simulink model "sim_magne_lev"  (R2021a)
settings: Solver=FixedStepAuto  StartTime=0.0  StopTime=15.0  RelTol=1e-3
undefined symbols (not defined in the file or in its folder): National_Instruments, PCIe
libraries: sldrtlib x2
settings Model: SimulationMode=external  Creator=磁気浮上  LastModifiedBy=磁気浮上
settings SolverCC: AlgebraicLoopSolver=TrustRegion  DecoupledContinuousIntegration=on  MinimalZcImpactIntegration=on
settings DataIOCC: ReturnWorkspaceOutputs=off
settings DebuggingCC: SFMachineParentedDataDiag=warning  ArithmeticOperatorsInVariantConditions=warning
settings SFSimCC: SimUseLocalCustomCode=off  CustomCodeUndefinedFunction=UseInterfaceOnly
settings RTWCC: Description=Simulink Desktop Real-Time  SystemTargetFile=sldrt.tlc  TemplateMakefile=sldrt.tmf  RTWUseLocalCustomCode=off  RTWCompilerOptimization=on
settings CodeAppCC: MaxIdLength=95
settings SimulinkDesktopRealTimeCC: TargetPreCompLibLocation=C:\Program Files\MATLAB\R2021a\toolbox\sldrt\lib\win64

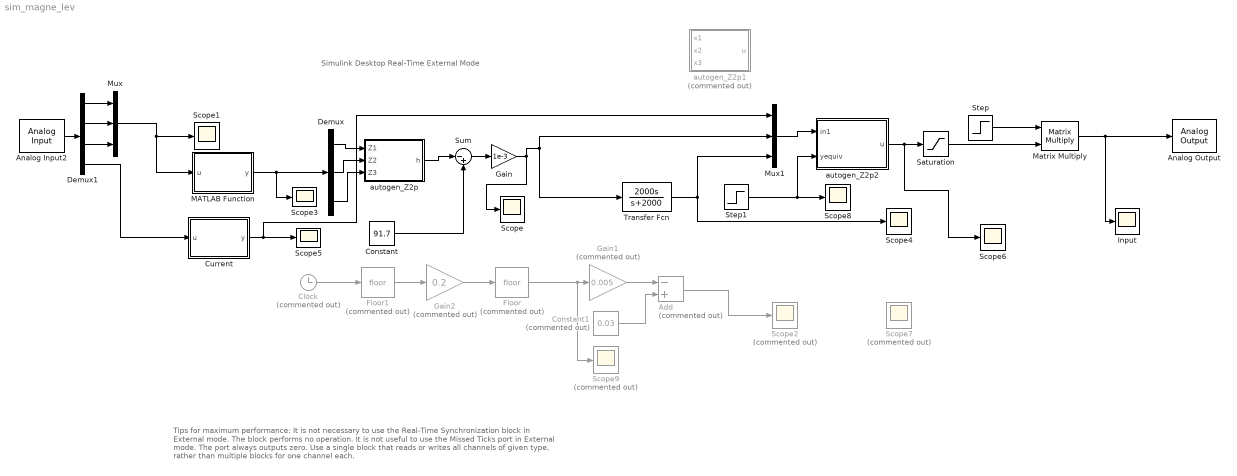
== system sim_magne_lev ==
  note: Simulink Desktop Real-Time External Mode
  note: Tips for maximum performance:
      |
      | It is not necessary to use the Real-Time Synchronization block in External mode. The block performs no operation.
      | It is not useful to use the Missed Ticks port in External mode. The port always outputs zero.
      | Use a single block that reads or writes all channels of given type, rather than multiple blocks for one channel each.
  Add : Sum  Commented=on  Inputs=-+
  Analog Input2 : sldrtlib/Analog Input  SampleTime=0.001  MaxMissedTicks=10  ShowMissedTicks=off  YieldWhenWaiting=off  DrvName=National_Instruments/PCIe-6361  DrvAddress=4294967295  DrvOptions=[0 0 0 0 0 0 0]  Channels=[1 2 3 5]  RangeMode=1  VoltRange=1  DataType=1
      settings: AttributesFormatString=National Instruments\nPCIe-6361 [auto]
  Analog Output : sldrtlib/Analog Output  SampleTime=0.001  MaxMissedTicks=10  ShowMissedTicks=off  YieldWhenWaiting=off  DrvName=National_Instruments/PCIe-6361  DrvAddress=4294967295  DrvOptions=[0 0 0 0 0 0 0]  Channels=1  RangeMode=1  VoltRange=1  InitialValue=[]  FinalValue=[]
      settings: AttributesFormatString=National Instruments\nPCIe-6361 [auto]
  Clock : Clock  Commented=on
  Constant : Constant  Value=91.7
  Constant1 : Constant  Commented=on  Value=0.03
  Current : MATLAB Function  TreatAsAtomicUnit=on
  Demux : Demux  Outputs=3
  Demux1 : Demux
  Floor : Rounding  Commented=on
  Floor1 : Rounding  Commented=on
  Gain : Gain  Gain=1e-3
  Gain1 : Gain  Commented=on  Gain=0.005
  Gain2 : Gain  Commented=on  Gain=0.2
  Input : Scope
  MATLAB Function : MATLAB Function  TreatAsAtomicUnit=on
  Matrix Multiply : Product  Multiplication=Matrix(*)
  Mux : Mux  Inputs=3
  Mux1 : Mux  Inputs=3
  Saturation : Saturate  UpperLimit=10  LowerLimit=-10
  Scope{,1,3..6,8} (7 alike) : Scope
  Scope2 : Scope  Commented=on
  Scope7 : Scope  Commented=on
  Scope9 : Scope  Commented=on
  Step : Step  Time=10  Before=1  After=0  SampleTime=0
  Step1 : Step  Time=5  Before=0.01  After=0.005  SampleTime=0
  Sum : Sum  Inputs=|-+
  Transfer Fcn : TransferFcn  Numerator=[2000 0]  Denominator=[1 2000]
  autogen_Z2p : MATLAB Function  TreatAsAtomicUnit=on
  autogen_Z2p1 : MATLAB Function  Commented=on  TreatAsAtomicUnit=on
  autogen_Z2p2 : MATLAB Function  TreatAsAtomicUnit=on
  wires:
  Step/1 -> Matrix Multiply/1
  Constant/1 -> Sum/2
  autogen_Z2p/1(h) -> Sum/1
  Matrix Multiply/1 -> Input/1, Analog Output/1
  Transfer Fcn/1 -> Mux1/3, Scope4/1
  MATLAB Function/1(y) -> Scope3/1, Demux/1
  Sum/1 -> Gain/1
  Demux/2 -> autogen_Z2p/2(Z2)
  Demux/1 -> autogen_Z2p/1(Z1)
  Saturation/1 -> Matrix Multiply/2
  autogen_Z2p2/1(u) -> Scope6/1, Saturation/1
  Demux/3 -> autogen_Z2p/3(Z3)
  Current/1(y) -> Mux1/1, Scope5/1
  Analog Input2/1 -> Demux1/1
  Demux1/1 -> Mux/1
  Demux1/4 -> Current/1(u)
  Demux1/3 -> Mux/3
  Demux1/2 -> Mux/2
  Mux/1 -> Scope1/1, MATLAB Function/1(u)
  Gain/1 -> Mux1/2, Transfer Fcn/1, Scope/1
  Mux1/1 -> autogen_Z2p2/1(in1)
  Constant1/1 -> Add/2
  Gain1/1 -> Add/1
  Add/1 -> Scope2/1
  Step1/1 -> Scope8/1, autogen_Z2p2/2(yequiv)
  Floor/1 -> Scope9/1, Gain1/1
  Gain2/1 -> Floor/1
  Floor1/1 -> Gain2/1
  Clock/1 -> Floor1/1

== matlab function sim_magne_lev/autogen_Z2p ==
  data: Z1 input; h output; Z2 input; Z3 input
function h = autogen_Z2p(Z1,Z2,Z3)
%#codegen

%    This function was generated by the Symbolic Math Toolbox version 8.7.
%    09-Feb-2022 18:15:15

t2 = Z1.^2;
t3 = Z1.^3;
t4 = Z2.^2;
t5 = Z2.^3;
t6 = Z3.^2;
t7 = Z3.^3;
t8 = Z1.*3.21e+2;
t9 = Z2.*1.297e+3;
t10 = Z3.*1.763e+3;
t11 = Z3.*2.576e+3;
t12 = Z2.*2.897e+3;
t13 = Z1.*3.06e+3;
t24 = Z2.*Z3.*1.0352122e+11;
t25 = Z2.*Z3.*2.0704244e+11;
t26 = Z1.*Z3.*9.135768e+10;
t27 = Z1.*Z3.*1.8271536e+11;
t28 = Z1.*Z2.*1.9595028e+11;
t29 = Z1.*Z2.*9.797514e+10;
t39 = Z1.*4.8999911281101e+13;
t41 = Z3.*4.7733218776365e+13;
t48 = Z2.*4.6020599945112e+13;
t56 = Z1.*Z3.*2.511664935e+13;
t57 = Z1.*1.42753730002578e+14;
t58 = Z2.*Z3.*5.124007469e+13;
t68 = Z1.*Z2.*4.264372839e+13;
t80 = Z1.*Z2.*1.7692425141e+14;
t82 = Z1.*Z3.*1.4293441815e+14;
t88 = Z2.*Z3.*2.2089361633e+14;
t14 = -t12;
t15 = -t13;
t16 = t2.*3.21e+6;
t17 = t4.*1.297e+7;
t18 = t6.*1.763e+7;
t19 = t6.*2.576e+7;
t20 = t4.*2.897e+7;
t21 = t2.*3.06e+7;
t30 = t4.*2.0149636e+11;
t31 = Z1.*t6.*4.567884e+10;
t32 = Z3.*t2.*4.567884e+10;
t33 = t2.*9.466641e+10;
t34 = t3.*9.466641e+10;
t35 = -t24;
t36 = t2.*1.8933282e+11;
t37 = -t25;
t38 = -t26;
t40 = t6.*1.948789e+11;
t42 = Z2.*t6.*5.176061e+10;
t43 = Z3.*t4.*5.176061e+10;
t44 = t4.*1.0074818e+11;
t45 = t5.*1.0074818e+11;
t46 = -t27;
t47 = -t28;
t49 = t6.*9.743945e+10;
t50 = t7.*9.743945e+10;
t51 = Z1.*t4.*4.898757e+10;
t52 = Z2.*t2.*4.898757e+10;
t53 = -t29;
t54 = Z2.*t3.*3.21e+10;
t55 = Z3.*t3.*3.21e+10;
t59 = Z1.*t7.*2.576e+11;
t60 = Z2.*t7.*2.576e+11;
t61 = Z1.*t7.*1.763e+11;
t62 = Z2.*t7.*1.763e+11;
t63 = Z1.*t5.*1.297e+11;
t64 = Z3.*t5.*1.297e+11;
t65 = Z2.*Z3.*t2.*4.66e+10;
t66 = Z2.*t3.*3.06e+11;
t67 = Z3.*t3.*3.06e+11;
t69 = Z1.*t5.*2.897e+11;
t70 = Z3.*t5.*2.897e+11;
t72 = t2.*1.699491663e+13;
t73 = Z1.*Z3.*t4.*4.823e+11;
t74 = Z2.*Z3.*t2.*5.473e+11;
t75 = Z1.*Z2.*t6.*4.357e+11;
t76 = Z1.*Z3.*t4.*2.255e+11;
t77 = -t58;
t79 = t2.*3.388018887e+13;
t84 = t4.*t6.*4.66e+10;
t86 = t6.*4.584717173e+13;
t87 = Z1.*Z2.*t6.*3.218e+11;
t91 = t4.*8.912494397e+13;
t92 = t2.*t6.*4.823e+11;
t93 = t4.*t6.*5.473e+11;
t94 = t2.*t4.*4.357e+11;
t96 = t2.*t6.*2.255e+11;
t98 = -t80;
t99 = t6.*9.788848349e+13;
t103 = t2.*t4.*3.218e+11;
t104 = -t88;
t105 = t4.*1.1408216305e+14;
t110 = t2.*2.85507460005156e+18;
t22 = -t20;
t23 = -t21;
t71 = -t55;
t78 = -t60;
t81 = -t62;
t83 = -t63;
t85 = -t66;
t89 = -t70;
t90 = -t73;
t95 = -t76;
t97 = -t79;
t100 = t8+t11+t14;
t101 = -t86;
t102 = -t87;
t106 = -t92;
t107 = -t96;
t108 = t9+t10+t15;
t109 = -t103;
t117 = t30+t36+t37+t40+t46+t47+1.42753730002578e+14;
t118 = t33+t35+t38+t44+t49+t53+7.1376865001289e+13;
t111 = t16+t19+t22-2.275477497e+9;
t112 = t17+t18+t23+3.0399800799e+10;
t119 = 1.0./t118;
t120 = 1.0./t117;
t113 = t111.^2;
t114 = t112.^2;
t115 = t100.*t111;
t116 = t108.*t112;
t121 = t110+t113+t114-2.569567140046404e+21;
t122 = t57+t115+t116;
t123 = t122.^2;
t125 = t118.*t121;
t124 = t123.*1.0e+4;
t126 = -t125;
t127 = t124+t126;
t128 = sqrt(t127);
t129 = t128./1.0e+2;
t130 = Z1.*t128.*3.799498679230342e-3;
t131 = Z1.*t128.*3.621952011976588e-2;
t132 = Z2.*t128.*1.535186849520796e-2;
t133 = Z3.*t128.*2.086765162455792e-2;
t134 = Z3.*t128.*3.049068098971141e-2;
t135 = Z2.*t128.*3.429017966894175e-2;
mt1 = [(t119.*(t61+t64+t65+t67+t72+t75+t77+t81+t82+t83+t84+t85+t90+t94+t98+t101+t105+t106+t130+t134-t135+1.922433295028705e+16))./2.0e+2,(t119.*(t61+t64+t65+t67+t72+t75+t77+t81+t82+t83+t84+t85+t90+t94+t98+t101+t105+t106-t130-t134+t135+1.922433295028705e+16))./2.0e+2,(t119.*(t54-t55+t56+t59-t60+t68+t69+t74+t89+t91+t93+t95+t97+t99+t102+t104+t107+t109+t131-t132-t133+3.556391874974202e+16))./2.0e+2];
mt2 = [(t119.*(t54+t56+t59+t68+t69+t71+t74+t78+t89+t91+t93+t95+t97+t99+t102+t104+t107+t109-t131+t132+t133+3.556391874974202e+16))./2.0e+2,t120.*(-t31-t32+t34+t39+t41-t42-t43+t45+t48+t50-t51-t52+t129)+3.0e+1,-t120.*(t31+t32-t34-t39-t41+t42+t43-t45-t48-t50+t51+t52+t129)+3.0e+1];
pv = reshape([mt1,mt2],2,3);

if pv(1,3)>0
    h=pv(1,3);
else
    h=pv(2,3);
end

== matlab function sim_magne_lev/autogen_Z2p1 ==
  data: x1 input; u output; x2 input; x3 input
function u = autogen_Z2p(x1,x2,x3)
%#codegen

%    This function was generated by the Symbolic Math Toolbox version 8.7.
%    06-May-2022 18:13:36

t2 = x1.^2;
t3 = 1.0./x1;
t4 = 1.0./x2;
t7 = x2+6.31e-2;
t5 = t4.^2;
t6 = t4.*(4.7e+1./1.0e+3);
t9 = t4.*1.73e-2;
t10 = 1.0./t7;
t8 = asinh(t6);
t11 = t10.^2;
t12 = asinh(t9);
t14 = t10.*(4.7e+1./1.0e+3);
t16 = t10.*1.73e-2;
t13 = -t12;
t15 = asinh(t14);
t17 = asinh(t16);
t18 = -t17;
t19 = t8+t13;
t20 = t19.*x2;
t21 = t15+t18;
t22 = t7.*t21;
t23 = -t22;
t24 = t20+t23;
t25 = t24.^2;
t26 = 1.0./t25;
et1 = t2.*t25.*2.964891883886256e+6;
et2 = t2.*t24.*x3.*(-t15+t17+t19+t7.*(t11.*1.0./sqrt(t11.*2.209e-3+1.0).*(4.7e+1./1.0e+3)-t11.*1.0./sqrt(t11.*2.9929e-4+1.0).*1.73e-2)-x2.*(t5.*1.0./sqrt(t5.*2.209e-3+1.0).*(4.7e+1./1.0e+3)-t5.*1.0./sqrt(t5.*2.9929e-4+1.0).*1.73e-2)).*(-2.962084221117424e+5);
u = t3.*t26.*(et1+et2).*1.94273525834272e-6+t3.*t26.*(x2.*1.0e+3+x3.*3.0e+2-t2.*t25.*4.443126331676137e+6+2.69e+2).*1.94273525834272e-6;

== matlab function sim_magne_lev/Current ==
  data: u input; y output
function y = fcn(u)
%u:バイポーラ電源の出力値（V）（電流を観測）、y:バイポーラ電源が流している電流(A)
    %出力電圧値が距離に変換されます。
    
%{ 
坂田（追記）
    装置から電流を観測している。
    実際の値とずれが生じているので補正をかけている
%}
    y=(3.01/6.23)*u;

== matlab function sim_magne_lev/autogen_Z2p2 ==
  data: in1 input; u output; yequiv input
function u = autogen_Z2p(in1,yequiv)
%#codegen

%    This function was generated by the Symbolic Math Toolbox version 8.7.
%    22-Jun-2022 16:39:22

x1 = in1(1,:);
x2 = in1(2,:);
x3 = in1(3,:);
t2 = x1.^2;
t3 = 1.0./x1;
t4 = 1.0./x2;
t6 = x2+2.77e-2;
t5 = t4.^2;
t7 = t4.*4.92e-2;
t8 = t4.*2.17e-2;
t9 = 1.0./t6;
t10 = t9.^2;
t11 = asinh(t7);
t12 = asinh(t8);
t14 = t9.*4.92e-2;
t15 = t9.*2.17e-2;
t13 = -t12;
t16 = asinh(t14);
t17 = asinh(t15);
t18 = -t17;
t19 = t11+t13;
t20 = t19.*x2;
t21 = t16+t18;
t22 = t6.*t21;
t23 = -t22;
t24 = t20+t23;
t25 = t24.^2;
t26 = 1.0./t25;
et1 = t3.*t26.*(t2.*t25.*6.397640088747686e+6-t2.*t24.*x3.*(-t16+t17+t19+t6.*(t10.*1.0./sqrt(t10.*2.42064e-3+1.0).*4.92e-2-t10.*1.0./sqrt(t10.*4.7089e-4+1.0).*2.17e-2)-x2.*(t5.*1.0./sqrt(t5.*2.42064e-3+1.0).*4.92e-2-t5.*1.0./sqrt(t5.*4.7089e-4+1.0).*2.17e-2)).*6.391581717451524e+5);
et2 = 9.003319849346977e-7;
u = et1.*et2+t3.*t26.*(x2.*1.0e+3+x3.*3.0e+2-yequiv.*1.0e+3-t2.*t25.*9.587372576177285e+6+2.94e+2).*9.003319849346977e-7;

== matlab function sim_magne_lev/MATLAB Function ==
  data: u input; y output
function y = fcn(u)
%u:光学センサの出力(V)、y:光学センサの出力PV値(mm)
    %出力スケーリングを行っています(フリーレンジ)。（光学センサの設定10,P.4-27）
    %PV値範囲を0～-50、出力電圧範囲を-5～5としているので、以下の式に従って
    %電圧値が距離に変換されます。
    y=(u-5*ones(3,1))*(-5);
% y = u;
